simulink model "DF_Stage4"  (R2015a)
settings: Solver=ode45  StartTime=0.0  StopTime=1e-3  RelTol=1e-3
libraries: dsparch4 x12
settings Model: Creator=John  LastModifiedBy=John

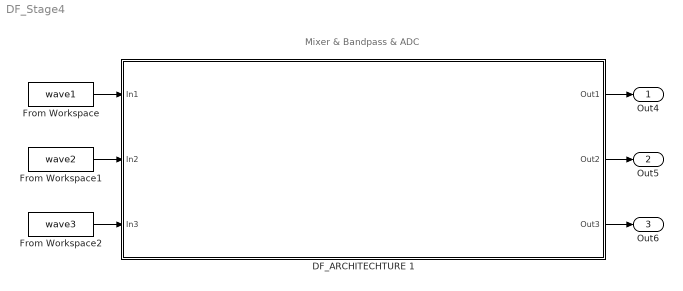
== system DF_Stage4 ==
  note: Mixer & Bandpass & ADC
  DF_ARCHITECHTURE 1 : Subsystem
  From Workspace : FromWorkspace  VariableName=wave1  SampleTime=0
  From Workspace1 : FromWorkspace  VariableName=wave2  SampleTime=0
  From Workspace2 : FromWorkspace  VariableName=wave3  SampleTime=0
  Out4 : Outport
  Out5 : Outport  Port=2
  Out6 : Outport  Port=3
  wires:
  From Workspace1/1 -> DF_ARCHITECHTURE 1/2(In2)
  From Workspace/1 -> DF_ARCHITECHTURE 1/1(In1)
  From Workspace2/1 -> DF_ARCHITECHTURE 1/3(In3)
  DF_ARCHITECHTURE 1/1(Out1) -> Out4/1
  DF_ARCHITECHTURE 1/2(Out2) -> Out5/1
  DF_ARCHITECHTURE 1/3(Out3) -> Out6/1

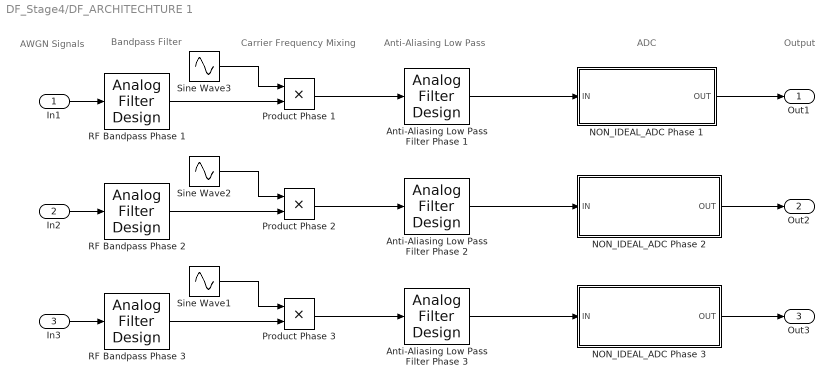
== system DF_Stage4/DF_ARCHITECHTURE 1 ==
  note: Anti-Aliasing Low Pass
  note: Carrier Frequency Mixing
  note: Output
  note: ADC
  note: Bandpass Filter
  note: AWGN Signals
  In1 : Inport
  In2 : Inport  Port=2
  In3 : Inport  Port=3
  Anti-Aliasing Low Pass Filter Phase 1 : dsparch4/Analog Filter Design  method=Butterworth  filttype=Lowpass  N=8  Wlo=2*pi*40e6  Whi=80  Rp=2  Rs=40
  Anti-Aliasing Low Pass Filter Phase 2 : dsparch4/Analog Filter Design  method=Butterworth  filttype=Lowpass  N=8  Wlo=2*pi*40e6  Whi=80  Rp=2  Rs=40
  Anti-Aliasing Low Pass Filter Phase 3 : dsparch4/Analog Filter Design  method=Butterworth  filttype=Lowpass  N=8  Wlo=2*pi*40e6  Whi=80  Rp=2  Rs=40
  NON_IDEAL_ADC Phase 1 : Subsystem
  NON_IDEAL_ADC Phase 2 : Subsystem
  NON_IDEAL_ADC Phase 3 : Subsystem
  Product Phase 1 : Product
  Product Phase 2 : Product
  Product Phase 3 : Product
  "RF Bandpass Phase 1 " : dsparch4/Analog Filter Design  method=Butterworth  filttype=Bandpass  N=8  Wlo=2*pi*5e6  Whi=2*pi*25e6  Rp=2  Rs=40
  RF Bandpass Phase 3 : dsparch4/Analog Filter Design  method=Butterworth  filttype=Bandpass  N=8  Wlo=2*pi*5e6  Whi=2*pi*25e6  Rp=2  Rs=40
  "RF Bandpass Phase 2 " : dsparch4/Analog Filter Design  method=Butterworth  filttype=Bandpass  N=8  Wlo=2*pi*5e6  Whi=2*pi*25e6  Rp=2  Rs=40
  Sine Wave1 : Sin  Frequency=20e6  Phase=pi/2  SampleTime=0
  Sine Wave2 : Sin  Frequency=15e6  Phase=pi/2  SampleTime=0
  Sine Wave3 : Sin  Frequency=2*pi*10e6  Phase=pi/2  SampleTime=0
  Out1 : Outport
  Out2 : Outport  Port=2
  Out3 : Outport  Port=3
  wires:
  In2/1 -> "RF Bandpass Phase 2 "/1
  In1/1 -> "RF Bandpass Phase 1 "/1
  NON_IDEAL_ADC Phase 1/1("OUT ") -> Out1/1
  NON_IDEAL_ADC Phase 2/1("OUT ") -> Out2/1
  NON_IDEAL_ADC Phase 3/1("OUT ") -> Out3/1
  In3/1 -> RF Bandpass Phase 3/1
  "RF Bandpass Phase 1 "/1 -> Product Phase 1/2
  "RF Bandpass Phase 2 "/1 -> Product Phase 2/2
  RF Bandpass Phase 3/1 -> Product Phase 3/2
  Product Phase 3/1 -> Anti-Aliasing Low Pass Filter Phase 3/1
  Product Phase 2/1 -> Anti-Aliasing Low Pass Filter Phase 2/1
  Product Phase 1/1 -> Anti-Aliasing Low Pass Filter Phase 1/1
  Anti-Aliasing Low Pass Filter Phase 3/1 -> NON_IDEAL_ADC Phase 3/1(IN)
  Anti-Aliasing Low Pass Filter Phase 2/1 -> NON_IDEAL_ADC Phase 2/1(IN)
  Anti-Aliasing Low Pass Filter Phase 1/1 -> NON_IDEAL_ADC Phase 1/1(IN)
  Sine Wave3/1 -> Product Phase 1/1
  Sine Wave2/1 -> Product Phase 2/1
  Sine Wave1/1 -> Product Phase 3/1

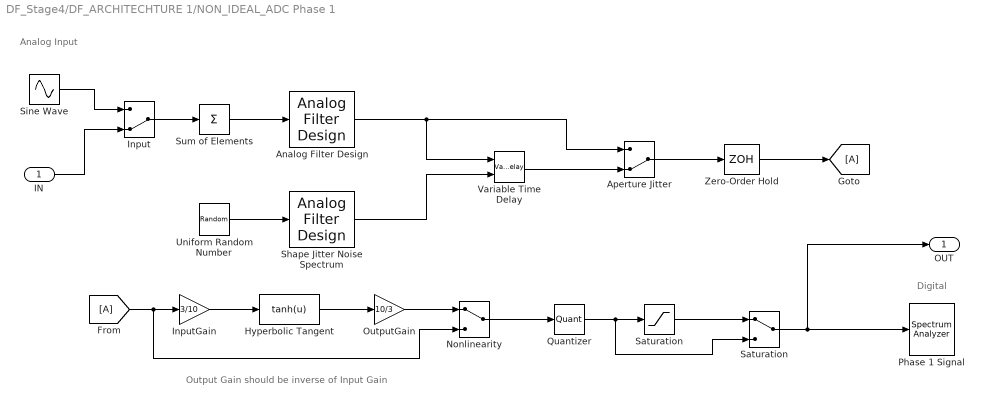
== system DF_Stage4/DF_ARCHITECHTURE 1/NON_IDEAL_ADC Phase 1 ==
  note: Output Gain should be inverse of Input Gain
  note: Digital
  note: Analog
      | Input
  IN : Inport
  Analog Filter Design : dsparch4/Analog Filter Design  method=Butterworth  filttype=Lowpass  N=8  Wlo=2*pi*40e6  Whi=80  Rp=2  Rs=40
  Aperture Jitter : ManualSwitch  CurrentSetting=0
  "Hyperbolic Tangent " : Fcn  Expr=tanh(u)
  "Input " : ManualSwitch  CurrentSetting=0
  InputGain : Gain  Gain=3/10
  "Nonlinearity " : ManualSwitch
  "OutputGain " : Gain  Gain=10/3
  Phase 1 Signal : SpectrumAnalyzer
  Quantizer : Quantizer  QuantizationInterval=2^-10
  Saturation : Saturate
  "Saturation " : ManualSwitch
  "Shape Jitter Noise Spectrum " : dsparch4/Analog Filter Design  method=Butterworth  filttype=Lowpass  N=3  Wlo=2*pi*10e+06  Whi=80  Rp=2  Rs=40
  Sine Wave : Sin  Amplitude=.25  Frequency=2*pi*[20 22]*1e6  SampleTime=0
  Sum of Elements : Sum  Inputs=+
  Uniform Random Number : UniformRandomNumber  Minimum=0  Maximum=5e-9  Seed=1234  SampleTime=0
  Variable Time Delay : VariableTransportDelay  MaximumDelay=30e-9  ZeroDelay=on  TransDelayFeedthrough=on
  Zero-Order Hold : ZeroOrderHold  SampleTime=1/80e6
  "OUT " : Outport
  wires:
  [A] -> InputGain/1, "Nonlinearity "/2
  Sine Wave/1 -> "Input "/1
  Analog Filter Design/1 -> Variable Time Delay/1, Aperture Jitter/1
  "OutputGain "/1 -> "Nonlinearity "/1
  Variable Time Delay/1 -> Aperture Jitter/2
  "Nonlinearity "/1 -> Quantizer/1
  "Saturation "/1 -> "OUT "/1, Phase 1 Signal/1
  "Input "/1 -> Sum of Elements/1
  IN/1 -> "Input "/2
  Quantizer/1 -> Saturation/1, "Saturation "/2
  Aperture Jitter/1 -> Zero-Order Hold/1
  InputGain/1 -> "Hyperbolic Tangent "/1
  "Hyperbolic Tangent "/1 -> "OutputGain "/1
  Saturation/1 -> "Saturation "/1
  Zero-Order Hold/1 -> [A]
  "Shape Jitter Noise Spectrum "/1 -> Variable Time Delay/2
  Uniform Random Number/1 -> "Shape Jitter Noise Spectrum "/1
  Sum of Elements/1 -> Analog Filter Design/1

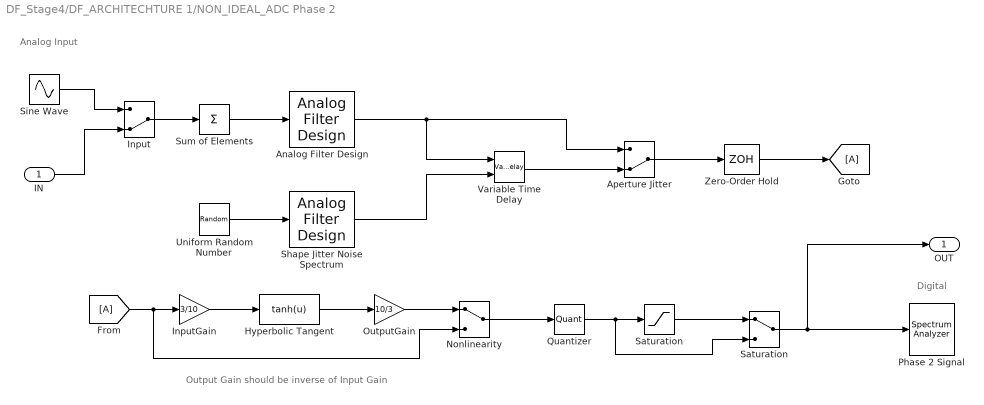
== system DF_Stage4/DF_ARCHITECHTURE 1/NON_IDEAL_ADC Phase 2 ==
  note: Output Gain should be inverse of Input Gain
  note: Digital
  note: Analog
      | Input
  IN : Inport
  Analog Filter Design : dsparch4/Analog Filter Design  method=Butterworth  filttype=Lowpass  N=8  Wlo=2*pi*40e6  Whi=80  Rp=2  Rs=40
  Aperture Jitter : ManualSwitch  CurrentSetting=0
  "Hyperbolic Tangent " : Fcn  Expr=tanh(u)
  "Input " : ManualSwitch  CurrentSetting=0
  InputGain : Gain  Gain=3/10
  "Nonlinearity " : ManualSwitch
  "OutputGain " : Gain  Gain=10/3
  Phase 2 Signal : SpectrumAnalyzer
  Quantizer : Quantizer  QuantizationInterval=2^-10
  Saturation : Saturate
  "Saturation " : ManualSwitch
  "Shape Jitter Noise Spectrum " : dsparch4/Analog Filter Design  method=Butterworth  filttype=Lowpass  N=3  Wlo=2*pi*10e+06  Whi=80  Rp=2  Rs=40
  Sine Wave : Sin  Amplitude=.25  Frequency=2*pi*[20 22]*1e6  SampleTime=0
  Sum of Elements : Sum  Inputs=+
  Uniform Random Number : UniformRandomNumber  Minimum=0  Maximum=5e-9  Seed=1234  SampleTime=0
  Variable Time Delay : VariableTransportDelay  MaximumDelay=30e-9  ZeroDelay=on  TransDelayFeedthrough=on
  Zero-Order Hold : ZeroOrderHold  SampleTime=1/80e6
  "OUT " : Outport
  wires:
  [A] -> InputGain/1, "Nonlinearity "/2
  Sine Wave/1 -> "Input "/1
  Analog Filter Design/1 -> Variable Time Delay/1, Aperture Jitter/1
  "OutputGain "/1 -> "Nonlinearity "/1
  Variable Time Delay/1 -> Aperture Jitter/2
  "Nonlinearity "/1 -> Quantizer/1
  "Saturation "/1 -> "OUT "/1, Phase 2 Signal/1
  "Input "/1 -> Sum of Elements/1
  IN/1 -> "Input "/2
  Quantizer/1 -> Saturation/1, "Saturation "/2
  Aperture Jitter/1 -> Zero-Order Hold/1
  InputGain/1 -> "Hyperbolic Tangent "/1
  "Hyperbolic Tangent "/1 -> "OutputGain "/1
  Saturation/1 -> "Saturation "/1
  Zero-Order Hold/1 -> [A]
  "Shape Jitter Noise Spectrum "/1 -> Variable Time Delay/2
  Uniform Random Number/1 -> "Shape Jitter Noise Spectrum "/1
  Sum of Elements/1 -> Analog Filter Design/1

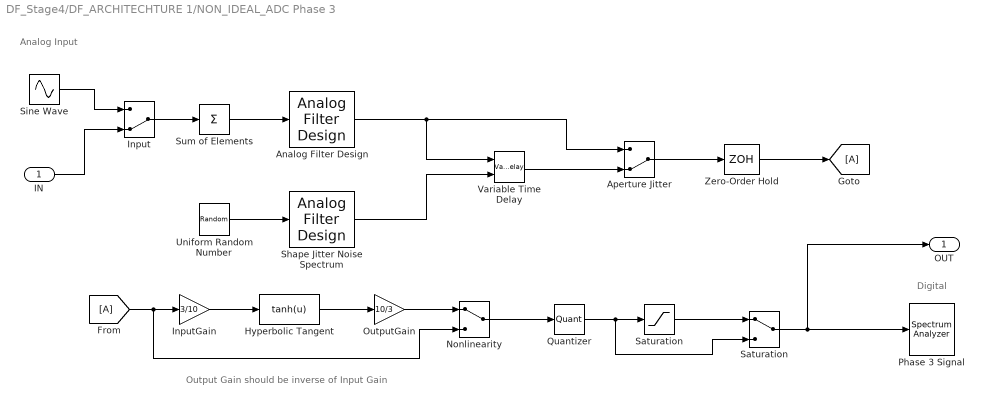
== system DF_Stage4/DF_ARCHITECHTURE 1/NON_IDEAL_ADC Phase 3 ==
  note: Output Gain should be inverse of Input Gain
  note: Digital
  note: Analog
      | Input
  IN : Inport
  Analog Filter Design : dsparch4/Analog Filter Design  method=Butterworth  filttype=Lowpass  N=8  Wlo=2*pi*40e6  Whi=80  Rp=2  Rs=40
  Aperture Jitter : ManualSwitch  CurrentSetting=0
  "Hyperbolic Tangent " : Fcn  Expr=tanh(u)
  "Input " : ManualSwitch  CurrentSetting=0
  InputGain : Gain  Gain=3/10
  "Nonlinearity " : ManualSwitch
  "OutputGain " : Gain  Gain=10/3
  Phase 3 Signal : SpectrumAnalyzer
  Quantizer : Quantizer  QuantizationInterval=2^-10
  Saturation : Saturate
  "Saturation " : ManualSwitch
  "Shape Jitter Noise Spectrum " : dsparch4/Analog Filter Design  method=Butterworth  filttype=Lowpass  N=3  Wlo=2*pi*10e+06  Whi=80  Rp=2  Rs=40
  Sine Wave : Sin  Amplitude=.25  Frequency=2*pi*[20 22]*1e6  SampleTime=0
  Sum of Elements : Sum  Inputs=+
  Uniform Random Number : UniformRandomNumber  Minimum=0  Maximum=5e-9  Seed=1234  SampleTime=0
  Variable Time Delay : VariableTransportDelay  MaximumDelay=30e-9  ZeroDelay=on  TransDelayFeedthrough=on
  Zero-Order Hold : ZeroOrderHold  SampleTime=1/80e6
  "OUT " : Outport
  wires:
  [A] -> InputGain/1, "Nonlinearity "/2
  Sine Wave/1 -> "Input "/1
  Analog Filter Design/1 -> Variable Time Delay/1, Aperture Jitter/1
  "OutputGain "/1 -> "Nonlinearity "/1
  Variable Time Delay/1 -> Aperture Jitter/2
  "Nonlinearity "/1 -> Quantizer/1
  "Saturation "/1 -> "OUT "/1, Phase 3 Signal/1
  "Input "/1 -> Sum of Elements/1
  IN/1 -> "Input "/2
  Quantizer/1 -> Saturation/1, "Saturation "/2
  Aperture Jitter/1 -> Zero-Order Hold/1
  InputGain/1 -> "Hyperbolic Tangent "/1
  "Hyperbolic Tangent "/1 -> "OutputGain "/1
  Saturation/1 -> "Saturation "/1
  Zero-Order Hold/1 -> [A]
  "Shape Jitter Noise Spectrum "/1 -> Variable Time Delay/2
  Uniform Random Number/1 -> "Shape Jitter Noise Spectrum "/1
  Sum of Elements/1 -> Analog Filter Design/1
